simulink model "SensorTest_2018a"  (R2018a)
settings: Solver=FixedStepAuto  StartTime=0.0  StopTime=60  FixedStep=Ts  RelTol=1e-3  EnableMultiTasking=on
InitFcn:
  | run('../model.m');
  | run('sensortest_hpf_load.m')
values from neighbouring files (symbols this model uses):
  ah = (tau_h/Ts)/(1 + (tau_h/Ts))    [sensortest_hpf_load.m]
undefined symbols (not defined in the file or in its folder): DiscIntNeverNeededParam, Ts
libraries: legoev3lib x1
settings Model: SimulationMode=external  ExtModeTrigDuration=2  Creator=thh206  LastModifiedBy=thh206
settings SolverCC: PositivePriorityOrder=on
settings OptimizationCC: EnhancedBackFolding=on  PassReuseOutputArgsAs=Individual arguments  MaxStackSize=64  OptimizeBlockOrder=speed  DifferentSizesBufferReuse=on  OptimizationCustomize=off
settings DebuggingCC: ParameterTunabilityLossMsg=error
settings HardwareCC: ProdBitPerPointer=32  ProdBitPerSizeT=32  ProdBitPerPtrDiffT=32  ProdLargestAtomicInteger=Long  ProdWordSize=32  ProdHWDeviceType=ARM Compatible->ARM 9
settings SFSimCC: MATLABDynamicMemAlloc=off
settings RTWCC: SystemTargetFile=ert.tlc  HardwareBoard=LEGO MINDSTORMS EV3  TLCOptions="-aInlineSetEventsForThisBaseRateFcn=TLC_FALSE -aSuppressMultiTaskScheduler=TLC_FALSE  -aRateBasedStepFcn=0"  TemplateMakefile=ert_default_tmf  GenerateReport=on  Toolchain=Sourcery G++ Lite v2009q3  IncludeHyperlinkInReport=on  LaunchReport=on  GenerateTraceInfo=on  GenerateTraceReport=on  GenerateTraceReportSl=on  GenerateTraceReportSf=on  GenerateTraceReportEml=on
settings CodeAppCC: ForceParamTrailComments=on  IgnoreCustomStorageClasses=off  OperatorAnnotations=on  SimulinkDataObjDesc=on  SFDataObjDesc=on  InsertBlockDesc=on
settings ERTTargetCC: SupportContinuousTime=on  SupportVariableSizeSignals=on

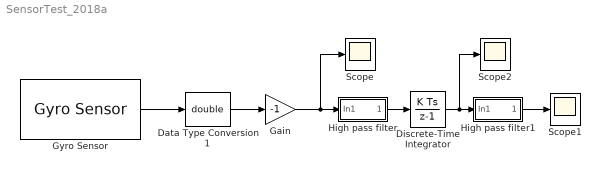
== system SensorTest_2018a ==
  Data Type Conversion1 : DataTypeConversion  OutDataTypeStr=double
  Discrete-Time Integrator : DiscreteIntegrator  SampleTime=Ts  ICPrevOutput=DiscIntNeverNeededParam  ICPrevScaledInput=DiscIntNeverNeededParam
  Gain : Gain  Gain=-1
  Gyro Sensor : legoev3lib/Gyro Sensor  portNumber=2  sampleTime=Ts
      settings: SourceProductName=Simulink Support Package for LEGO MINDSTORMS EV3 Hardware  SourceProductBaseCode=LEGOEV3
  High pass filter : Subsystem
  High pass filter1 : Subsystem
  Scope : Scope
  Scope1 : Scope
  Scope2 : Scope
  wires:
  Data Type Conversion1/1 -> Gain/1
  Gyro Sensor/1 -> Data Type Conversion1/1
  Gain/1 -> High pass filter/1(In1), Scope/1
  High pass filter/1(Out1) -> Discrete-Time Integrator/1
  Discrete-Time Integrator/1 -> Scope2/1, High pass filter1/1(In1)
  High pass filter1/1(Out1) -> Scope1/1

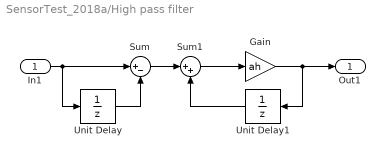
== system SensorTest_2018a/High pass filter ==
  In1 : Inport
  Gain : Gain  Gain=ah
  Sum : Sum  Inputs=|+-
  Sum1 : Sum  Inputs=|++
  Unit Delay : UnitDelay  SampleTime=-1  HasFrameUpgradeWarning=on
  Unit Delay1 : UnitDelay  SampleTime=-1  HasFrameUpgradeWarning=on
  Out1 : Outport
  wires:
  In1/1 -> Unit Delay/1, Sum/1
  Unit Delay/1 -> Sum/2
  Sum/1 -> Sum1/1
  Unit Delay1/1 -> Sum1/2
  Sum1/1 -> Gain/1
  Gain/1 -> Unit Delay1/1, Out1/1

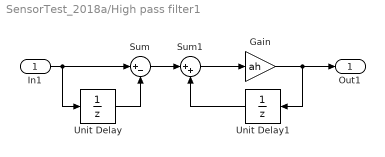
== system SensorTest_2018a/High pass filter1 ==
  In1 : Inport
  Gain : Gain  Gain=ah
  Sum : Sum  Inputs=|+-
  Sum1 : Sum  Inputs=|++
  Unit Delay : UnitDelay  SampleTime=-1  HasFrameUpgradeWarning=on
  Unit Delay1 : UnitDelay  SampleTime=-1  HasFrameUpgradeWarning=on
  Out1 : Outport
  wires:
  In1/1 -> Unit Delay/1, Sum/1
  Unit Delay/1 -> Sum/2
  Sum/1 -> Sum1/1
  Unit Delay1/1 -> Sum1/2
  Sum1/1 -> Gain/1
  Gain/1 -> Unit Delay1/1, Out1/1
